simulink model "Demo"  (Simulink 6.2)
settings: Solver=ode45  StartTime=0.0  StopTime=10.0  RelTol=1e-3
settings Model: Creator=suarezjl  LastModifiedBy=suarezjl
settings DataIOCC: SignalLoggingName=sigsOut
settings HardwareCC: TargetUnknown=on

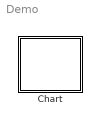
== system Demo ==
  Chart : Stateflow chart

== stateflow chart Chart ==
  state StopStateMachines
    \\Aquateen\ControlBasisModule\HP3JCAgent\StateMachine.ManualSignal()
    \\Aquateen\ControlBasisModule\ForceSensor\StateMachine.ManualSignal()
  state Start Motoman
    \\Aquateen\ControlBasisModule\HP3JCAgent\StateMachine.LoadSM()
    \\Aquateen\ControlBasisModule\HP3JCAgent\StateMachine.Start()
    \\Aquateen\ControlBasisModule\DemoStateMachine.Wait(100)
  state Start FT Sensor
    \\Aquateen\ControlBasisModule\ForceSensor\StateMachine.LoadSM()
    \\Aquateen\ControlBasisModule\ForceSensor\StateMachine.Start()
    \\Aquateen\ControlBasisModule\DemoStateMachine.Wait(100)
  (default) -> Start FT Sensor : Start
  Start Motoman -> StopStateMachines : Signal="End"
  Start FT Sensor -> Start Motoman : Always
